simulink model "Scalar_Calculator_Task"  (R2021a)
settings: Solver=FixedStepDiscrete  StartTime=0.0  StopTime=10.0  RelTol=1e-3
libraries: simulink x3
settings Model: Creator=Dell  LastModifiedBy=Dell
settings OptimizationCC: DefaultParameterBehavior=Inlined  EnhancedBackFolding=on  PassReuseOutputArgsAs=Individual arguments  ZeroExternalMemoryAtStartup=off  ZeroInternalMemoryAtStartup=off  OptimizeBlockOrder=speed  DifferentSizesBufferReuse=on  OptimizationCustomize=off  EfficientTunableParamExpr=on
settings DebuggingCC: ParameterTunabilityLossMsg=error
settings SFSimCC: MATLABDynamicMemAlloc=off
settings RTWCC: SystemTargetFile=ert.tlc  GenCodeOnly=on  TemplateMakefile=ert_default_tmf  GenerateReport=on  IncludeHyperlinkInReport=on  LaunchReport=on  GenerateTraceInfo=on
settings CodeAppCC: ForceParamTrailComments=on  IgnoreCustomStorageClasses=off  OperatorAnnotations=on  SimulinkDataObjDesc=on  SFDataObjDesc=on  InsertBlockDesc=on
settings ERTTargetCC: TargetLangStandard=C99 (ISO)  GenerateSampleERTMain=on  InlinedParameterPlacement=NonHierarchical  ERTCustomFileTemplate=example_file_process.tlc

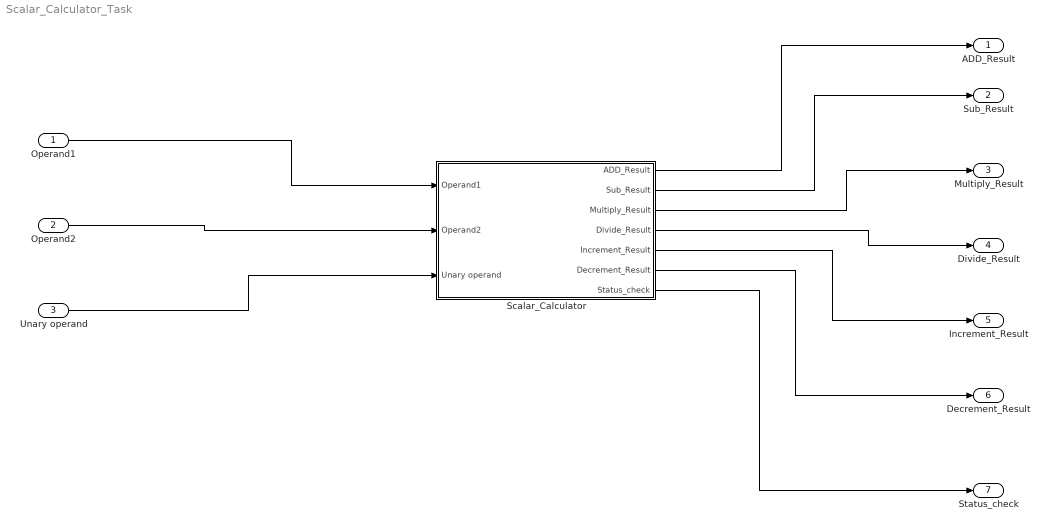
== system Scalar_Calculator_Task ==
  Operand1 : Inport  OutDataTypeStr=uint8
  Operand2 : Inport  Port=2  OutDataTypeStr=uint8
  Unary operand : Inport  Port=3  OutDataTypeStr=uint8
  Scalar_Calculator : Subsystem
  ADD_Result : Outport
  Sub_Result : Outport  Port=2
  Multiply_Result : Outport  Port=3
  Divide_Result : Outport  Port=4
  Increment_Result : Outport  Port=5
  Decrement_Result : Outport  Port=6
  Status_check : Outport  Port=7  OutDataTypeStr=boolean
  wires:
  Operand1/1 -> Scalar_Calculator/1(Operand1)
  Operand2/1 -> Scalar_Calculator/2(Operand2)
  Unary operand/1 -> Scalar_Calculator/3(Unary operand)
  Scalar_Calculator/1(ADD_Result) -> ADD_Result/1
  Scalar_Calculator/2(Sub_Result) -> Sub_Result/1
  Scalar_Calculator/3(Multiply_Result) -> Multiply_Result/1
  Scalar_Calculator/4(Divide_Result) -> Divide_Result/1
  Scalar_Calculator/5(Increment_Result) -> Increment_Result/1
  Scalar_Calculator/6(Decrement_Result) -> Decrement_Result/1
  Scalar_Calculator/7(Status_check) -> Status_check/1

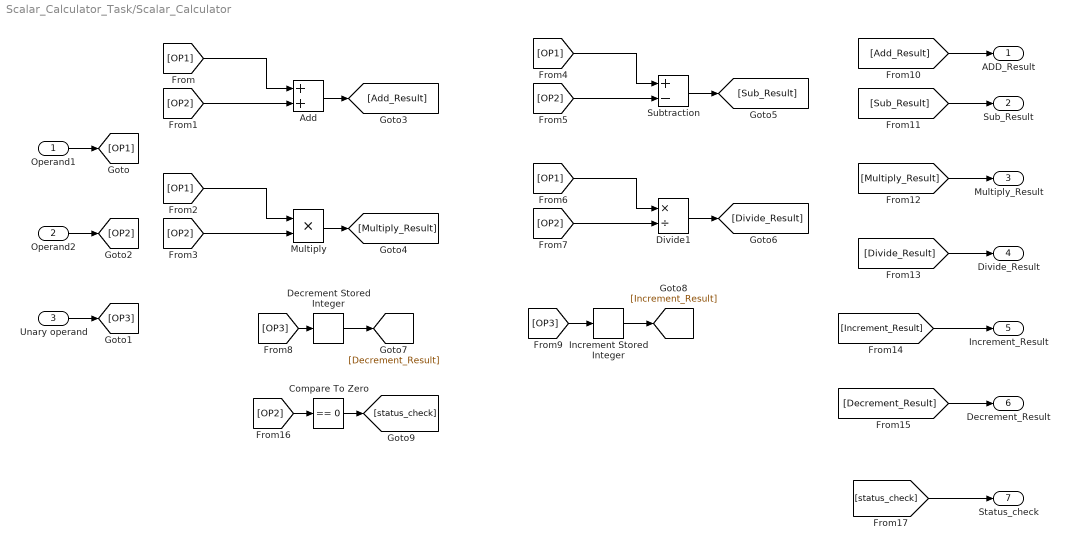
== system Scalar_Calculator_Task/Scalar_Calculator ==
  Operand1 : Inport  OutDataTypeStr=uint8
  Operand2 : Inport  Port=2  OutDataTypeStr=uint8
  Unary operand : Inport  Port=3  OutDataTypeStr=uint8
  Add : Sum
  Compare To Zero : simulink/Logic and Bit Operations/Compare To Zero  relop===  OutDataTypeStr=boolean
  Decrement Stored Integer : simulink/Additional Math & Discrete/Additional Math: Increment - Decrement/Decrement Stored Integer
      settings: SourceProductBaseCode=SL
  Divide1 : Product  Inputs=*/
  Increment Stored Integer : simulink/Additional Math & Discrete/Additional Math: Increment - Decrement/Increment Stored Integer
  Multiply : Product
  Subtraction : Sum  Inputs=+-
  ADD_Result : Outport
  Sub_Result : Outport  Port=2
  Multiply_Result : Outport  Port=3
  Divide_Result : Outport  Port=4
  Increment_Result : Outport  Port=5
  Decrement_Result : Outport  Port=6
  Status_check : Outport  Port=7  OutDataTypeStr=boolean
  wires:
  [OP2] -> Divide1/2
  [Sub_Result] -> Sub_Result/1
  [OP2] -> Add/2
  [Add_Result] -> ADD_Result/1
  [OP1] -> Divide1/1
  Operand1/1 -> [OP1]
  [OP3] -> Decrement Stored Integer/1
  Compare To Zero/1 -> [status_check]
  [Decrement_Result] -> Decrement_Result/1
  Operand2/1 -> [OP2]
  Increment Stored Integer/1 -> [Increment_Result]
  [Increment_Result] -> Increment_Result/1
  Subtraction/1 -> [Sub_Result]
  [OP2] -> Compare To Zero/1
  Decrement Stored Integer/1 -> [Decrement_Result]
  [OP1] -> Add/1
  [OP1] -> Multiply/1
  [OP2] -> Multiply/2
  [OP1] -> Subtraction/1
  [OP2] -> Subtraction/2
  Multiply/1 -> [Multiply_Result]
  [Multiply_Result] -> Multiply_Result/1
  Unary operand/1 -> [OP3]
  Add/1 -> [Add_Result]
  [OP3] -> Increment Stored Integer/1
  Divide1/1 -> [Divide_Result]
  [Divide_Result] -> Divide_Result/1
  [status_check] -> Status_check/1
